simulink model "thermodynamic_properties_ideal_gas_test"  (R2017b)
settings: Solver=VariableStepAuto  StartTime=0.0  StopTime=0  RelTol=1e-3
undefined symbols (not defined in the file or in its folder): P, rho, T, v
libraries: thermochemical x16
settings Model: Creator=ferru  LastModifiedBy=fferrucc

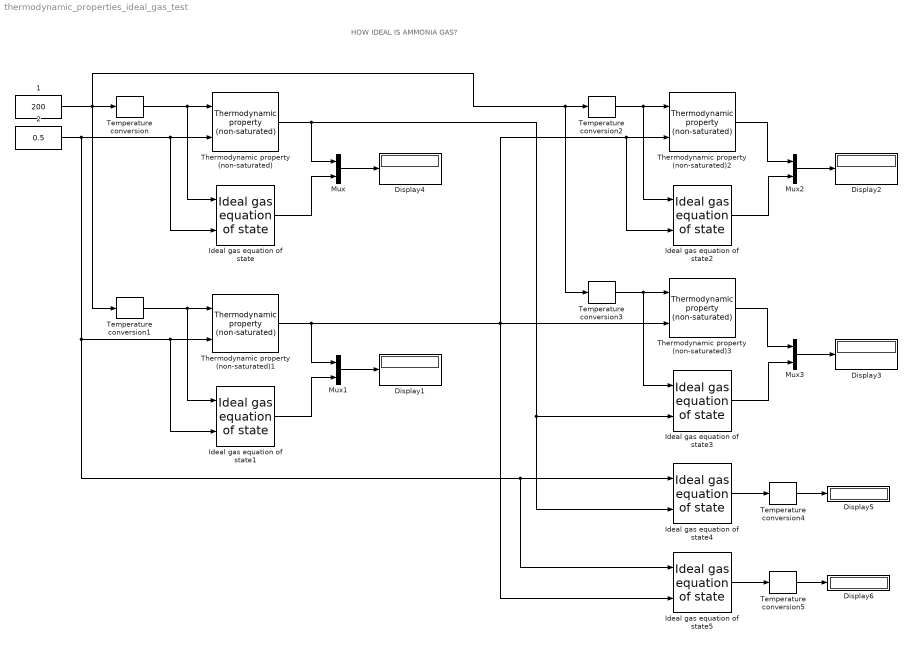
== system thermodynamic_properties_ideal_gas_test ==
  note: HOW IDEAL IS AMMONIA GAS?
  1 : Constant  Value=200
  2 : Constant  Value=0.5
  Display{1..6} (6 alike) : Display
  Ideal gas equation of state : thermochemical/Thermodynamic fluid properties/Ideal gas equation of state  sel=v(T,P)  R=8.3145  Pa_to_bar=1e-5  bar_to_Pa=1e5
      settings: SourceProductName=@ Thermochemical
  Ideal gas equation of state1 : thermochemical/Thermodynamic fluid properties/Ideal gas equation of state  sel=rho(T,P)  R=8.3145  Pa_to_bar=1e-5  bar_to_Pa=1e5
      settings: SourceProductName=@ Thermochemical
  Ideal gas equation of state2 : thermochemical/Thermodynamic fluid properties/Ideal gas equation of state  sel=P(T,rho)  R=8.3145  Pa_to_bar=1e-5  bar_to_Pa=1e5
      settings: SourceProductName=@ Thermochemical
  Ideal gas equation of state3 : thermochemical/Thermodynamic fluid properties/Ideal gas equation of state  sel=P(T,v)  R=8.3145  Pa_to_bar=1e-5  bar_to_Pa=1e5
      settings: SourceProductName=@ Thermochemical
  Ideal gas equation of state4 : thermochemical/Thermodynamic fluid properties/Ideal gas equation of state  sel=T(P,v)  R=8.3145  Pa_to_bar=1e-5  bar_to_Pa=1e5
      settings: SourceProductName=@ Thermochemical
  Ideal gas equation of state5 : thermochemical/Thermodynamic fluid properties/Ideal gas equation of state  sel=T(P,rho)  R=8.3145  Pa_to_bar=1e-5  bar_to_Pa=1e5
      settings: SourceProductName=@ Thermochemical
  Mux{,1..3} (4 alike) : Mux  Inputs=2
  Temperature conversion{,1..3} (4 alike) : thermochemical/Conversions/Temperature conversion  sel=°C --> K
      settings: SourceProductName=@ Thermochemical
  Temperature conversion4 : thermochemical/Conversions/Temperature conversion  sel=K --> °C
      settings: SourceProductName=@ Thermochemical
  Temperature conversion5 : thermochemical/Conversions/Temperature conversion  sel=K --> °C
      settings: SourceProductName=@ Thermochemical
  Thermodynamic property (non-saturated) : thermochemical/Thermodynamic fluid properties/Thermodynamic  property (non-saturated)  sel=v(T,P)  fluid=nh3_v4  reciprocVar=+1  lookup2D_BreakPoint1=nh3_v4.no_sat.T_P_indep.var_indep.T  lookup2D_BreakPoint2=nh3_v4.no_sat.T_P_indep.var_indep.P  lookup2D_Data=nh3_v4.no_sat.T_P_indep.var_dep.rho_molar
      settings: SourceProductName=@ Thermochemical
  Thermodynamic property (non-saturated)1 : thermochemical/Thermodynamic fluid properties/Thermodynamic  property (non-saturated)  sel=rho(T,P)  fluid=nh3_v4  reciprocVar=-1  lookup2D_BreakPoint1=nh3_v4.no_sat.T_P_indep.var_indep.T  lookup2D_BreakPoint2=nh3_v4.no_sat.T_P_indep.var_indep.P  lookup2D_Data=nh3_v4.no_sat.T_P_indep.var_dep.rho_molar
      settings: SourceProductName=@ Thermochemical
  Thermodynamic property (non-saturated)2 : thermochemical/Thermodynamic fluid properties/Thermodynamic  property (non-saturated)  sel=P(T,rho)  fluid=nh3_v4  reciprocVar=-1  lookup2D_BreakPoint1=nh3_v4.no_sat.T_rho_indep.var_indep.T  lookup2D_BreakPoint2=nh3_v4.no_sat.T_rho_indep.var_indep.rho_molar  lookup2D_Data=nh3_v4.no_sat.T_rho_indep.var_dep.P
      settings: SourceProductName=@ Thermochemical
  Thermodynamic property (non-saturated)3 : thermochemical/Thermodynamic fluid properties/Thermodynamic  property (non-saturated)  sel=P(T,rho)  fluid=nh3_v4  reciprocVar=-1  lookup2D_BreakPoint1=nh3_v4.no_sat.T_rho_indep.var_indep.T  lookup2D_BreakPoint2=nh3_v4.no_sat.T_rho_indep.var_indep.rho_molar  lookup2D_Data=nh3_v4.no_sat.T_rho_indep.var_dep.P
      settings: SourceProductName=@ Thermochemical
  wires:
  Temperature conversion/1 -> Ideal gas equation of state/1, Thermodynamic property (non-saturated)/1
  Ideal gas equation of state/1 -> Mux/2
  Mux/1 -> Display4/1
  Mux1/1 -> Display1/1
  Ideal gas equation of state1/1 -> Mux1/2
  2/1 -> Ideal gas equation of state4/1, Ideal gas equation of state5/1, Ideal gas equation of state1/2, Thermodynamic property (non-saturated)1/2, Ideal gas equation of state/2, Thermodynamic property (non-saturated)/2
  Temperature conversion1/1 -> Thermodynamic property (non-saturated)1/1, Ideal gas equation of state1/1
  Mux2/1 -> Display2/1
  Ideal gas equation of state2/1 -> Mux2/2
  Thermodynamic property (non-saturated)2/1 -> Mux2/1
  Temperature conversion2/1 -> Thermodynamic property (non-saturated)2/1, Ideal gas equation of state2/1
  1/1 -> Temperature conversion3/1, Temperature conversion2/1, Temperature conversion1/1, Temperature conversion/1
  Temperature conversion3/1 -> Ideal gas equation of state3/1, Thermodynamic property (non-saturated)3/1
  Thermodynamic property (non-saturated)/1 -> Ideal gas equation of state4/2, Ideal gas equation of state3/2, Mux/1
  Thermodynamic property (non-saturated)3/1 -> Mux3/1
  Ideal gas equation of state3/1 -> Mux3/2
  Mux3/1 -> Display3/1
  Ideal gas equation of state4/1 -> Temperature conversion4/1
  Thermodynamic property (non-saturated)1/1 -> Mux1/1, Thermodynamic property (non-saturated)2/2, Ideal gas equation of state2/2, Ideal gas equation of state5/2, Thermodynamic property (non-saturated)3/2
  Ideal gas equation of state5/1 -> Temperature conversion5/1
  Temperature conversion4/1 -> Display5/1
  Temperature conversion5/1 -> Display6/1
